simulink model "ABS_system"  (R2021a)
settings: Solver=VariableStepAuto  StartTime=0.0  StopTime=60  RelTol=1e-3
model workspace (MAT data in the model file):
  J = 1.13
  R = 0.33
  V0 = 27.78
  g = 9.81
  m = 342
settings Model: OrderedModelArguments=off  Creator=91839  LastModifiedBy=91839

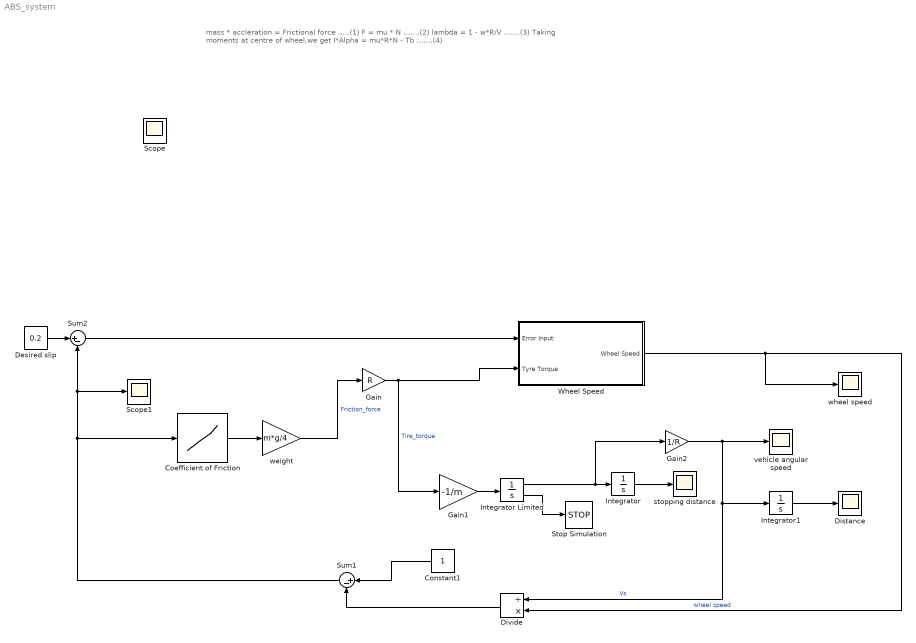
== system ABS_system ==
  note: mass * accleration = Frictional force .....(1)
      |
      | F = mu * N .......(2)
      |
      | lambda = 1 - w*R/V .......(3)
      |
      | Taking moments at centre of wheel,we get
      |
      | I*Alpha = mu*R*N - Tb .......(4)
  Coefficient of Friction : Lookup_n-D  NumberOfTableDimensions=1  BreakpointsForDimension1=[0,0.05,0.1,0.15,0.2,0.25,0.3,0.35,0.4,0.45,0.5,0.55,0.6,0.65,0.7,0.75,0.8,0.85,0.9,0.95,1]  Table=[0,0.4,0.8,0.97,1,0.98,0.96,0.94,0.92,0.9,0.88,0.885,0.83,0.81,0.79,0.77,0.75,0.73,0.72,0.71,0.70]  InternalRulePriority=Speed  RndMeth=Simplest  InputSameDT=on
  Constant1 : Constant
  Desired slip : Constant  Value=0.2
  Distance : Scope
  Divide : Product  Inputs=/*
  Gain : Gain  Gain=R
  Gain1 : Gain  Gain=-1/m
  Gain2 : Gain  Gain=1/R
  Integrator : Integrator
  Integrator Limited : Integrator  InitialCondition=V0  LimitOutput=on  UpperSaturationLimit=1000  LowerSaturationLimit=0  ShowSaturationPort=on
  Integrator1 : Integrator
  Scope1 : Scope
  Stop Simulation : Stop
  Sum1 : Sum  Inputs=|+-
  Sum2 : Sum  Inputs=|+-
  Wheel Speed : Subsystem
  stopping distance : Scope
  vehicle angular speed : Scope
  weight : Gain  Gain=m*g/4
  wheel speed : Scope
  Scope : Scope
  wires:
  Gain/1 -> Gain1/1, Wheel Speed/2(Tyre Torque)  "Tire_torque"
  Coefficient of Friction/1 -> weight/1
  weight/1 -> Gain/1  "Friction_force"
  Gain1/1 -> Integrator Limited/1
  Desired slip/1 -> Sum2/1
  Sum1/1 -> Coefficient of Friction/1, Sum2/2, Scope1/1
  Integrator/1 -> stopping distance/1
  Divide/1 -> Sum1/2
  Constant1/1 -> Sum1/1
  Sum2/1 -> Wheel Speed/1(Error Input)
  Wheel Speed/1(Wheel Speed) -> wheel speed/1, Divide/2  "wheel speed"
  Integrator Limited/2 -> Stop Simulation/1
  Gain2/1 -> vehicle angular speed/1, Integrator1/1, Divide/1  "Vs"
  Integrator Limited/1 -> Gain2/1, Integrator/1
  Integrator1/1 -> Distance/1

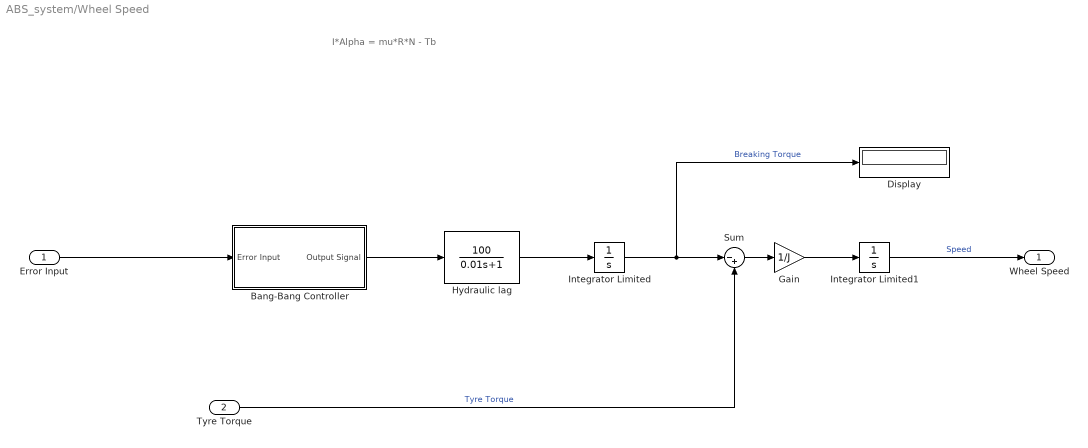
== system ABS_system/Wheel Speed ==
  note: I*Alpha = mu*R*N - Tb
  Error Input : Inport
  Tyre Torque : Inport  Port=2
  Bang-Bang Controller : Subsystem
  Display : Display
  Gain : Gain  Gain=1/J
  Hydraulic lag : TransferFcn  Numerator=[100]  Denominator=[0.01 1]
  Integrator Limited : Integrator  LimitOutput=on  UpperSaturationLimit=1000  LowerSaturationLimit=0
  Integrator Limited1 : Integrator  InitialCondition=V0/R  LimitOutput=on  UpperSaturationLimit=1000  LowerSaturationLimit=0
  Sum : Sum  Inputs=|-+
  Wheel Speed : Outport
  wires:
  Hydraulic lag/1 -> Integrator Limited/1
  Integrator Limited/1 -> Display/1, Sum/1  "Breaking Torque"
  Tyre Torque/1 -> Sum/2  "Tyre Torque"
  Sum/1 -> Gain/1
  Gain/1 -> Integrator Limited1/1
  Integrator Limited1/1 -> Wheel Speed/1  "Speed"
  Error Input/1 -> Bang-Bang Controller/1(Error Input)
  Bang-Bang Controller/1(Output Signal) -> Hydraulic lag/1

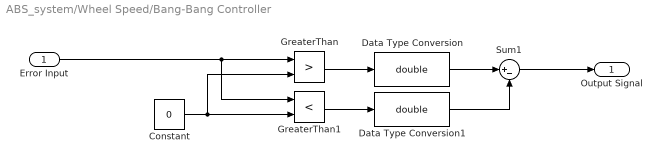
== system ABS_system/Wheel Speed/Bang-Bang Controller ==
  Error Input : Inport
  Constant : Constant  Value=0
  Data Type Conversion : DataTypeConversion  OutDataTypeStr=double  RndMeth=Zero
  Data Type Conversion1 : DataTypeConversion  OutDataTypeStr=double  RndMeth=Zero
  GreaterThan : RelationalOperator  Operator=>  OutDataTypeStr=boolean  RndMeth=Simplest
  GreaterThan1 : RelationalOperator  Operator=<  OutDataTypeStr=boolean  RndMeth=Simplest
  Sum1 : Sum  Inputs=|+-
  Output Signal : Outport
  wires:
  GreaterThan1/1 -> Data Type Conversion1/1
  Constant/1 -> GreaterThan/2, GreaterThan1/2
  Sum1/1 -> Output Signal/1
  Data Type Conversion1/1 -> Sum1/2
  GreaterThan/1 -> Data Type Conversion/1
  Data Type Conversion/1 -> Sum1/1
  Error Input/1 -> GreaterThan1/1, GreaterThan/1
